simulink model "final"  (R2024a)
settings: Solver=ode23t  StartTime=0.0  StopTime=1  RelTol=1e-6
model workspace (MAT data in the model file):
  Ts = 0.10201388834
undefined symbols (not defined in the file or in its folder): DiscIntNeverNeededParam, Ion, Lithium
libraries: spsIGBTDiodeLib x13, slpidlib x9, spsSeriesRLCBranchLib x7, spsCurrentMeasurementLib x6, spsThreePhaseSeriesRLCBranchLib x6, spsThreePhaseVIMeasurementLib x5, spsAlphaBetaZerotodq0Lib x4, spsGroundLib x3, spsPower3phInstantaneousLib x3, spsMosfetLib x2, simulink x2, spsdq0toabcLib x2
(part 3 of 3)

== matlab function final/SOC /MATLAB Function ==
  data: u input; y output
function y = fcn(u)

y = -u;

== matlab function final/MATLAB Function ==
  data: mode input; modeText output
function modeText = mode_to_text(mode)
% mode : entier venant de l'EMS

% Initialisation obligatoire (sécurité Simulink)
modeText = "Inconnu";

switch mode
    case 1
        modeText = "PV alimente charge";
    case 2
        modeText = "Charge batterie";
    case 3
        modeText = "Decharge batterie";
    case 4
        modeText = "Achat reseau";
    case 5
        modeText = "Mode Ilote";
    case 6
        modeText = "Vente reseau Et Charge batterie";
    case 7
        modeText = "Vente au reseau ";

    otherwise
        modeText = "Mode non defini";
end
